simulink model "LithiumBatteryChargerBlock"  (R2023a)
settings: Solver=ode1  StartTime=0.0  StopTime=7200  RelTol=1e-3
undefined symbols (not defined in the file or in its folder): Ion, Lithium
libraries: spsControlledCurrentSourceLib x2, spsBreakerLib x2, simulink x1, spsControlledVoltageSourceLib x1, spsBatteryLib x1, sps_lib x1
settings Model: Creator=Rodney Tan  LastModifiedBy=sandu
settings SolverCC: AlgebraicLoopSolver=TrustRegion
settings DataIOCC: ReturnWorkspaceOutputs=off
settings DebuggingCC: UnconnectedInputMsg=warning  UnconnectedOutputMsg=warning  UnconnectedLineMsg=warning  ArithmeticOperatorsInVariantConditions=warning
settings ModelReferenceCC: EnableRefExpFcnMdlSchedulingChecks=on
settings SFSimCC: SimUseLocalCustomCode=off  CustomCodeUndefinedFunction=UseInterfaceOnly
settings RTWCC: RTWUseLocalCustomCode=off

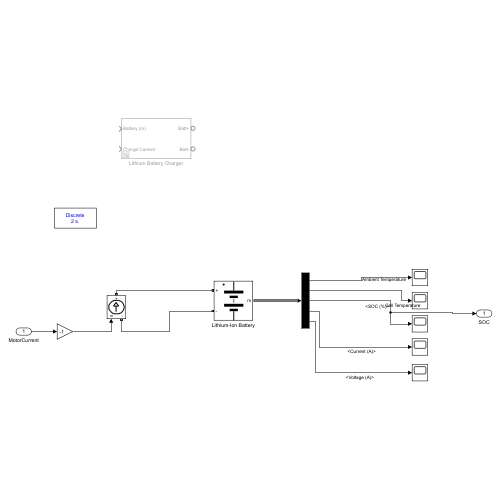
[thumbnail: Simulink's stored preview of the top-level diagram]
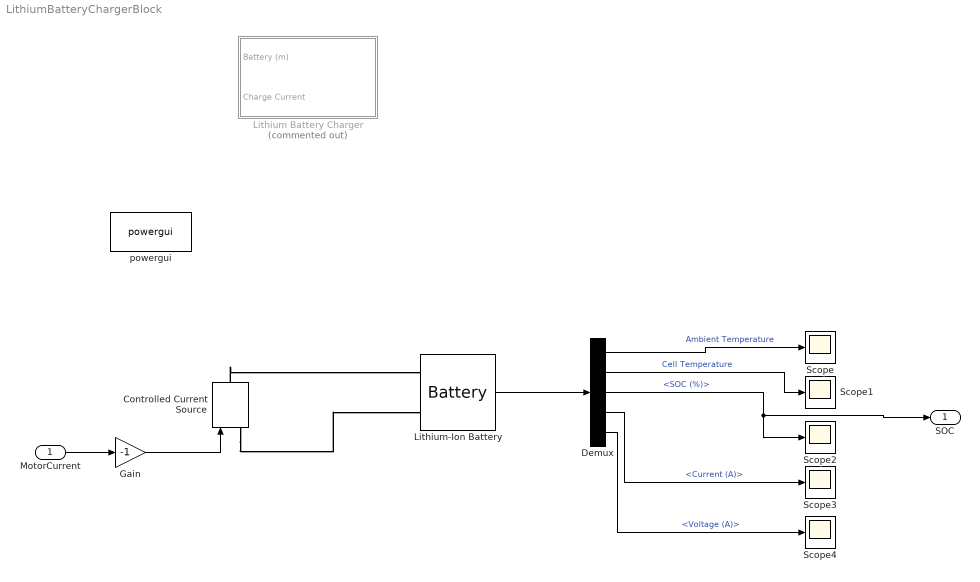
== system LithiumBatteryChargerBlock ==
  MotorCurrent : Inport
  Controlled Current Source : spsControlledCurrentSourceLib/Controlled Current Source  Initialize=on  Source_Type=AC  Amplitude=0  Phase=0  Frequency=0  Measurements=None
  Demux : Demux  Outputs=5
  Gain : Gain  Gain=-1
  Lithium Battery Charger : Subsystem  Commented=on  mask(Lithium Battery Charger){CV=4.3}
      mask prompts: CV "Saturation Charge Constant Voltage (V)"
      mask help:
      | Lithium Battery Charger Block Developed By Rodney Tan (PhD)
      | Version 1.00 (Aug 2019)
      |
      | This charger charge Lithium-Ion battery in two stages
      | This charger takes in charge current (A) from the input in (CC) Constant Current charging stage and switch to Saturation Charge (CV) Constant Voltage charging stage when the battery reaches the set constant voltage.
  Lithium-Ion Battery : spsBatteryLib/Battery  BatType=Lithium-Ion  ShowTempParam=off  ThermalPreset=no  ShowAgeParam=on  NomV=370  NomQ=300  SOC=100  Batt_Tr=20  PresetModel=on  MaxQ=300  MinV=277.5  FullV=430.6752  Dis_rate=130.4348  R=0.012333  Normal_OP=271.3043  expZone="[399.7428      14.73913]"  current=[1.2 0.6 0.3]  Units=Time  Tci=20  NomT=25  T2=0  MaxQ2=2.208  FullV2=3.45  Normal_OP2=2.8  expZone2="[3.22        0.23]"  Rca=0.6  ti=1000  Dp=0  Neq0=0  Tsim=1e6  Ta1=25  Qeol=5.4*0.9  Reol=0.013333*1.2  Char_age=[2.3478, 3]  Dis_age=[2.3478, 10]  N1=1500  N2=10500  N3=1000  N4=1400  Ta2=45  N5=950
      settings: LibrarySourceBlock=electricdrivelib/Extra Sources/Battery
  Scope{,1..4} (5 alike) : Scope
  powergui : sps_lib/powergui  Priority=1  SimulationMode=Discrete  SampleTime=2  frequency=60  Iterations=50  frequencyindice=0  Pbase=100e6  ErrMax=1e-4  UnitsV=kV  UnitsW=MW  buscounter=0  FunctionMessages=off  echomessages=off  EnableUseOfTLC=off  CurrentSourceSwitches=off  DisableSnubberDevices=off  DisableRonSwitches=off  DisableVfSwitches=off  DisplayEquations=off  AutomaticDiscreteSolvers=off  SolverType=Tustin/Backward Euler (TBE)  Interpol=off  ExternalGateDelay=off  methode=off  Ts=100  x0status=blocks  SPID=on  SwTol=0  HookPort=off  NonlinearTolerance=1e-4  nMaxIteration=100  ContinueOnMaxIteration=off  RestoreLinks=warning  ResistiveCurrentMeasurement=off  Frange=[0:2:500]  Ylog=off  Xlog=on  ShowGrid=off  save=off  variable=ZData  structure=0  ZoomFFT=off  StartTime=0.0  cycles=1  DisplayStyle=1  fundamental=60  FreqAxis=off  MaxFrequency=1000  frequencyindicesteady=1  RmsSteady=1  display=off
  SOC : Outport
  wires:
  MotorCurrent/1 -> Gain/1
  Lithium-Ion Battery/1 -> Demux/1
  Demux/1 -> Scope/1  "Ambient Temperature"
  Demux/2 -> Scope1/1  "Cell Temperature"
  Demux/3 -> Scope2/1, SOC/1  "<SOC (%)>"
  Gain/1 -> Controlled Current Source/1
  Demux/4 -> Scope3/1  "<Current (A)>"
  Demux/5 -> Scope4/1  "<Voltage (A)>"
  connections:
  Controlled Current Source/RConn1 -- Lithium-Ion Battery/LConn1
  Controlled Current Source/LConn1 -- Lithium-Ion Battery/LConn2

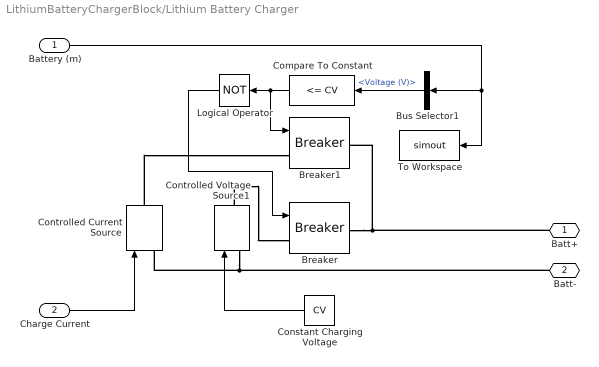
== system LithiumBatteryChargerBlock/Lithium Battery Charger ==
  Battery (m) : Inport
  Charge Current : Inport  Port=2
  Breaker : spsBreakerLib/Breaker  InitialState=0  SwitchingTimes="[1/60  5/60]"  External=on  BreakerResistance=0.01  SnubberResistance=10e6  SnubberCapacitance=inf  Measurements=None  MoreParameters=on  NoBreakLoop=off
  Breaker1 : spsBreakerLib/Breaker  InitialState=0  SwitchingTimes="[1/60  5/60]"  External=on  BreakerResistance=0.01  SnubberResistance=1e6  SnubberCapacitance=inf  Measurements=None  MoreParameters=on  NoBreakLoop=off
  Bus Selector1 : BusSelector  OutputSignals=Voltage (V)
  Compare To Constant : simulink/Logic and Bit Operations/Compare To Constant  relop=<=  const=CV  OutDataTypeStr=boolean
  Constant Charging Voltage : Constant  Value=CV
  Controlled Current Source : spsControlledCurrentSourceLib/Controlled Current Source  Initialize=on  Source_Type=DC  Amplitude=0  Phase=0  Frequency=0  Measurements=None
  Controlled Voltage Source1 : spsControlledVoltageSourceLib/Controlled Voltage Source  Initialize=on  Source_Type=DC  Amplitude=0  Phase=0  Frequency=0  Measurements=None
  Logical Operator : Logic  Operator=NOT  AllPortsSameDT=off  OutDataTypeStr=boolean
  To Workspace : ToWorkspace  VariableName=simout  SampleTime=-1
  Batt+ : PMIOPort  Side=Right
  Batt- : PMIOPort  Port=2  Side=Right
  wires:
  Bus Selector1/1 -> Compare To Constant/1  "<Voltage (V)>"
  Constant Charging Voltage/1 -> Controlled Voltage Source1/1
  Battery (m)/1 -> To Workspace/1, Bus Selector1/1
  Logical Operator/1 -> Breaker/1
  Compare To Constant/1 -> Logical Operator/1, Breaker1/1
  Charge Current/1 -> Controlled Current Source/1
  connections:
  Breaker/RConn1 -- Batt+/RConn1 -- Breaker1/RConn1
  Controlled Voltage Source1/RConn1 -- Breaker/LConn1
  Controlled Current Source/RConn1 -- Breaker1/LConn1
  Controlled Voltage Source1/LConn1 -- Batt-/RConn1 -- Controlled Current Source/LConn1
